simulink model "sim004"  (R2023b)
settings: Solver=FixedStepAuto  StartTime=0.0  StopTime=5  FixedStep=0.001  RelTol=1e-3  EnableMultiTasking=on
values from neighbouring files (symbols this model uses):
  a1 = 40    [FK.m]    (also in IK_Analytical.m = 0.04; IK_MDH.m = 0.04; IK_Position.m = 0.04; IK_Solver.m = 0.04)
  a2 = 275    [FK.m]    (also in IK_Analytical.m = 0.275; IK_MDH.m = 0.275; IK_Position.m = 0.275; IK_Solver.m = 0.275)
  a3 = 25    [FK.m]    (also in IK_Analytical.m = 0.025; IK_MDH.m = 0.025; IK_Position.m = 0.025; IK_Solver.m = 0.025)
  d1 = 342    [FK.m]    (also in IK_Analytical.m = 0.342; IK_MDH.m = 0.342; IK_Position.m = 0.342; IK_Solver.m = 0.342)
  d4 = 280    [FK.m]    (also in IK_Analytical.m = 0.28; IK_MDH.m = 0.28; IK_Position.m = 0.28; IK_Solver.m = 0.28)
  fc1 = 0    [set_mode_parameter.m]
  fc2 = 0    [set_mode_parameter.m]
  fc3 = 0    [set_mode_parameter.m]
  fc4 = 0    [set_mode_parameter.m]
  fc5 = 0    [set_mode_parameter.m]
  fc6 = 0    [set_mode_parameter.m]
  fv1 = 0    [set_mode_parameter.m]
  fv2 = 0    [set_mode_parameter.m]
  fv3 = 0    [set_mode_parameter.m]
  fv4 = 0    [set_mode_parameter.m]
  fv5 = 0    [set_mode_parameter.m]
  fv6 = 0    [set_mode_parameter.m]
  Ia1 = 0    [set_mode_parameter.m]
  Ia2 = 0    [set_mode_parameter.m]
  Ia3 = 0    [set_mode_parameter.m]
  Ia4 = 0    [set_mode_parameter.m]
  Ia5 = 0    [set_mode_parameter.m]
  Ia6 = 0    [set_mode_parameter.m]
  Ic111 = 0    [set_mode_parameter.m]
  Ic112 = 0    [set_mode_parameter.m]
  Ic113 = 0    [set_mode_parameter.m]
  Ic122 = 0    [set_mode_parameter.m]
  Ic123 = 0    [set_mode_parameter.m]
  Ic133 = 1.3676    [set_mode_parameter.m]
  Ic211 = 8.8194    [set_mode_parameter.m]
  Ic212 = 0    [set_mode_parameter.m]
  Ic213 = 0    [set_mode_parameter.m]
  Ic222 = 6.0549    [set_mode_parameter.m]
  Ic223 = 0    [set_mode_parameter.m]
  Ic233 = 0.9569    [set_mode_parameter.m]
  Ic311 = 0.0332    [set_mode_parameter.m]
  Ic312 = 0    [set_mode_parameter.m]
  Ic313 = 0    [set_mode_parameter.m]
  Ic322 = 1.8442    [set_mode_parameter.m]
  Ic323 = 0    [set_mode_parameter.m]
  Ic333 = 1.0560    (= 1.056)    [set_mode_parameter.m]
  Ic411 = 0.1448    [set_mode_parameter.m]
  Ic412 = 0    [set_mode_parameter.m]
  Ic413 = 0    [set_mode_parameter.m]
  Ic422 = 0.0015    [set_mode_parameter.m]
  Ic423 = 0    [set_mode_parameter.m]
  Ic433 = 0.0822    [set_mode_parameter.m]
  Ic511 = 0    [set_mode_parameter.m]
  Ic512 = 0    [set_mode_parameter.m]
  Ic513 = 0    [set_mode_parameter.m]
  Ic522 = 0.0121    [set_mode_parameter.m]
  Ic523 = 0    [set_mode_parameter.m]
  Ic533 = 0.0299    [set_mode_parameter.m]
  Ic611 = 0.0134    [set_mode_parameter.m]
  Ic612 = 0    [set_mode_parameter.m]
  Ic613 = 0    [set_mode_parameter.m]
  Ic622 = 0    [set_mode_parameter.m]
  Ic623 = 0    [set_mode_parameter.m]
  Ic633 = 0.0051    [set_mode_parameter.m]
  m = (c1*px + s1*py) - dt*(c1*ax + s1*ay) - a1    [IK_6DOF_Robot.m]    (also in IK_MDH.m = pwx_1 - a1; IK_MDH_Robot.m = rho - a1)
  m1 = 0.167    [set_mode_parameter.m]
  m2 = 1    [set_mode_parameter.m]
  m3 = 0.5    [set_mode_parameter.m]
  m4 = 0.333    [set_mode_parameter.m]
  m5 = 0.25    [set_mode_parameter.m]
  m6 = 0.2    [set_mode_parameter.m]
  mc11 = 0    [set_mode_parameter.m]
  mc12 = 0    [set_mode_parameter.m]
  mc13 = 0.2    [set_mode_parameter.m]
  mc21 = 0.1291    [set_mode_parameter.m]
  mc22 = 0    [set_mode_parameter.m]
  mc23 = 3.3117    [set_mode_parameter.m]
  mc31 = 1.6484    [set_mode_parameter.m]
  mc32 = 0    [set_mode_parameter.m]
  mc33 = 0.8748    [set_mode_parameter.m]
  mc41 = 0.3200    (= 0.32)    [set_mode_parameter.m]
  mc42 = 0.2324    [set_mode_parameter.m]
  mc43 = 0.7083    [set_mode_parameter.m]
  mc51 = 0.4574    [set_mode_parameter.m]
  mc52 = 0    [set_mode_parameter.m]
  mc53 = 0.6427    [set_mode_parameter.m]
  mc61 = 0.3200    (= 0.32)    [set_mode_parameter.m]
  mc62 = -0.0513    [set_mode_parameter.m]
  mc63 = 0.6417    [set_mode_parameter.m]
  N = size(waypoints, 2)    [run_trajectory.m]
  s = zc - d(1)    [inverse_kinematics_6dof.m]
  XB4 = SerialLink([L1 L2 L3 L4 L5 L6], 'name', 'XB4')    [Toolbox_Motheds_1.m]
undefined symbols (not defined in the file or in its folder): X, Y, Z
libraries: sm_lib x56, nesl_utility x31, simulink x2, simulink_extras x1
(part 1 of 2)
settings Model: Creator=Administrator  LastModifiedBy=jiehuang
settings SolverCC: AlgebraicLoopSolver=TrustRegion
settings DataIOCC: ReturnWorkspaceOutputs=off
settings OptimizationCC: LifeSpan=inf
settings DebuggingCC: UnconnectedInputMsg=warning  UnconnectedOutputMsg=warning  UnconnectedLineMsg=warning  SFUnexpectedBacktrackingDiag=warning  SFNoUnconditionalDefaultTransitionDiag=warning  ArithmeticOperatorsInVariantConditions=warning
settings ModelReferenceCC: EnableRefExpFcnMdlSchedulingChecks=on
settings SFSimCC: SimUseLocalCustomCode=off  CustomCodeUndefinedFunction=UseInterfaceOnly
settings RTWCC: RTWUseLocalCustomCode=off
settings CodeAppCC: StateflowObjectComments=on
settings GRTTargetCC: TargetLangStandard=C89/C90 (ANSI)
settings ConfigComp: CovMetricSettings=dw  CovSaveCumulativeToWorkspaceVar=on  CovSaveSingleToWorkspaceVar=on  CovExternalEMLEnable=off
settings SimscapeCC: SimscapeNormalizeSystem=off

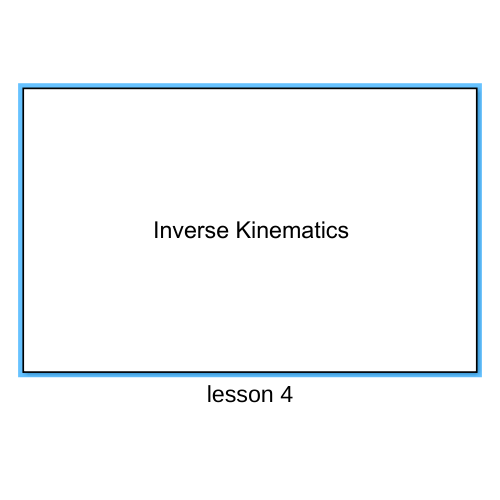
[thumbnail: Simulink's stored preview of the top-level diagram]
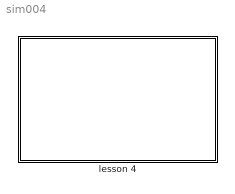
== system sim004 ==
  lesson 4 : Subsystem
      mask Display: disp('Inverse Kinematics')

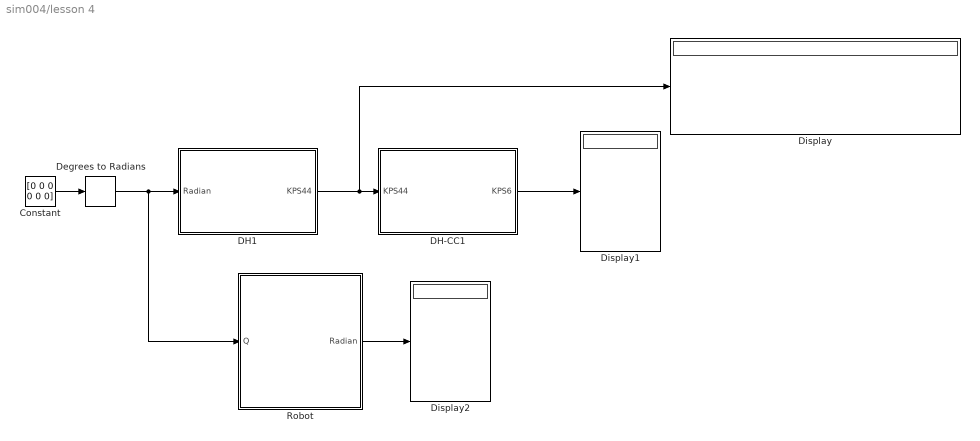
== system sim004/lesson 4 ==
  Constant : Constant  Value=[0 0 0 0 0 0]  VectorParams1D=off
  DH-CC1 : MATLAB Function  TreatAsAtomicUnit=on
  DH1 : MATLAB Function  TreatAsAtomicUnit=on
  Degrees to Radians : simulink_extras/Transformations/Degrees to Radians
  Display : Display
      settings: Decimation=16
  Display1 : Display
      settings: Decimation=6
  Display2 : Display
      settings: Decimation=6
  Robot : Subsystem
  wires:
  DH1/1(KPS44) -> Display/1, DH-CC1/1(KPS44)
  DH-CC1/1(KPS6) -> Display1/1
  Robot/1(Radian) -> Display2/1
  Constant/1 -> Degrees to Radians/1
  Degrees to Radians/1 -> Robot/1(Q), DH1/1(Radian)

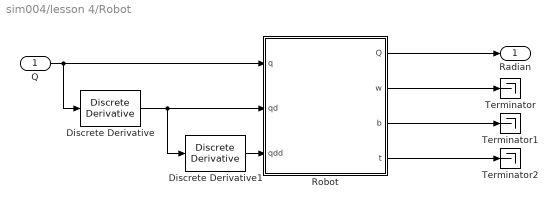
== system sim004/lesson 4/Robot ==
  Q : Inport
  Discrete Derivative : simulink/Discrete/Discrete Derivative  gainval=1.0  ICPrevScaledInput=0.0  OutMin=[]  OutMax=[]  OutDataType=fixdt(1, 16)  OutScaling=2^-10  DoSatur=off
  Discrete Derivative1 : simulink/Discrete/Discrete Derivative  gainval=1.0  ICPrevScaledInput=0.0  OutMin=[]  OutMax=[]  OutDataType=fixdt(1, 16)  OutScaling=2^-10  DoSatur=off
  Robot : Subsystem
  Terminator : Terminator
  Terminator1 : Terminator
  Terminator2 : Terminator
  Radian : Outport
  wires:
  Robot/1(Q) -> Radian/1
  Robot/2(w) -> Terminator/1
  Robot/3(b) -> Terminator1/1
  Robot/4(t) -> Terminator2/1
  Q/1 -> Discrete Derivative/1, Robot/1(q)
  Discrete Derivative/1 -> Discrete Derivative1/1, Robot/2(qd)
  Discrete Derivative1/1 -> Robot/3(qdd)

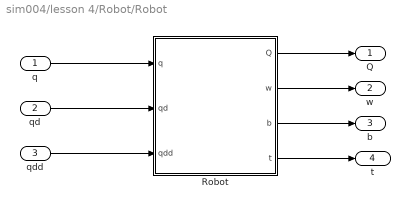
== system sim004/lesson 4/Robot/Robot ==
  q : Inport
  qd : Inport  Port=2
  qdd : Inport  Port=3
  Robot : Subsystem
  Q : Outport
  w : Outport  Port=2
  b : Outport  Port=3
  t : Outport  Port=4
  wires:
  Robot/1(Q) -> Q/1
  Robot/2(w) -> w/1
  Robot/3(b) -> b/1
  Robot/4(t) -> t/1
  q/1 -> Robot/1(q)
  qd/1 -> Robot/2(qd)
  qdd/1 -> Robot/3(qdd)

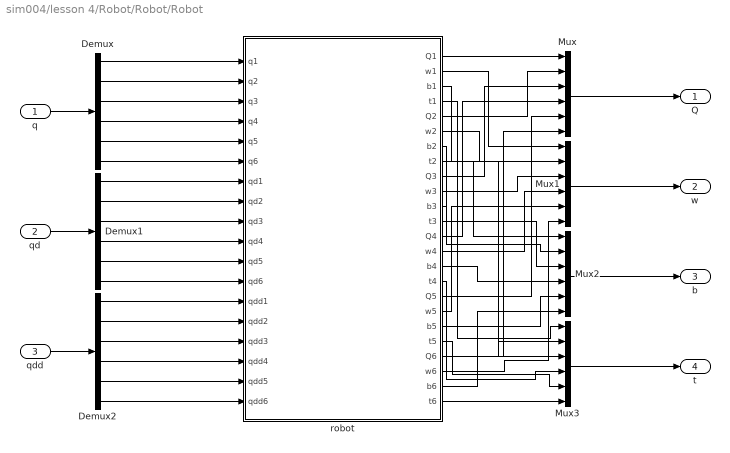
== system sim004/lesson 4/Robot/Robot/Robot ==
  q : Inport
  qd : Inport  Port=2
  qdd : Inport  Port=3
  Demux : Demux  Outputs=6
  Demux1 : Demux  Outputs=6
  Demux2 : Demux  Outputs=6
  Mux{,1..3} (4 alike) : Mux  Inputs=6
  robot : Subsystem
  Q : Outport
  w : Outport  Port=2
  b : Outport  Port=3
  t : Outport  Port=4
  wires:
  q/1 -> Demux/1
  robot/1(Q1) -> Mux/1
  robot/5(Q2) -> Mux/2
  robot/9(Q3) -> Mux/3
  robot/13(Q4) -> Mux/4
  robot/17(Q5) -> Mux/5
  robot/21(Q6) -> Mux/6
  robot/2(w1) -> Mux1/1
  robot/3(b1) -> Mux2/1
  robot/6(w2) -> Mux1/2
  robot/10(w3) -> Mux1/3
  robot/14(w4) -> Mux1/4
  robot/18(w5) -> Mux1/5
  robot/22(w6) -> Mux1/6
  robot/7(b2) -> Mux2/2
  robot/11(b3) -> Mux2/3
  robot/15(b4) -> Mux2/4
  robot/19(b5) -> Mux2/5
  robot/23(b6) -> Mux2/6
  robot/4(t1) -> Mux3/1
  robot/8(t2) -> Mux3/2
  robot/12(t3) -> Mux3/3
  robot/16(t4) -> Mux3/4
  robot/20(t5) -> Mux3/5
  robot/24(t6) -> Mux3/6
  Mux/1 -> Q/1
  Mux1/1 -> w/1
  Mux2/1 -> b/1
  Mux3/1 -> t/1
  Demux/1 -> robot/1(q1)
  Demux/2 -> robot/2(q2)
  Demux/3 -> robot/3(q3)
  Demux/4 -> robot/4(q4)
  Demux/5 -> robot/5(q5)
  Demux/6 -> robot/6(q6)
  Demux1/2 -> robot/8(qd2)
  Demux1/3 -> robot/9(qd3)
  Demux1/4 -> robot/10(qd4)
  Demux1/5 -> robot/11(qd5)
  Demux1/6 -> robot/12(qd6)
  Demux1/1 -> robot/7(qd1)
  qd/1 -> Demux1/1
  Demux2/2 -> robot/14(qdd2)
  Demux2/3 -> robot/15(qdd3)
  Demux2/4 -> robot/16(qdd4)
  Demux2/5 -> robot/17(qdd5)
  Demux2/6 -> robot/18(qdd6)
  Demux2/1 -> robot/13(qdd1)
  qdd/1 -> Demux2/1

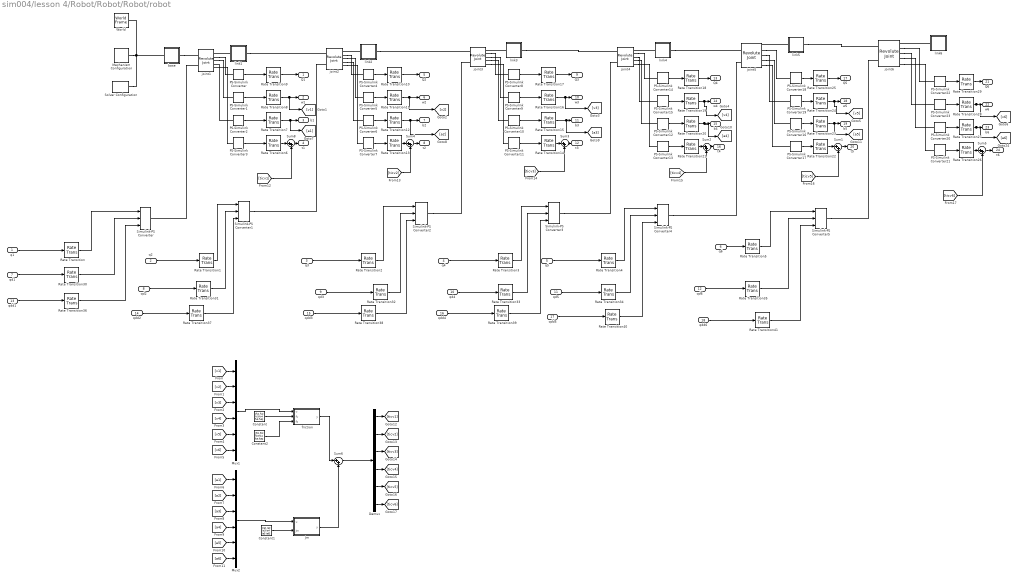
== system sim004/lesson 4/Robot/Robot/Robot/robot ==
  q1 : Inport
  q2 : Inport  Port=2
  q3 : Inport  Port=3
  q4 : Inport  Port=4
  q5 : Inport  Port=5
  q6 : Inport  Port=6
  qd1 : Inport  Port=7
  qd2 : Inport  Port=8
  qd3 : Inport  Port=9
  qd4 : Inport  Port=10
  qd5 : Inport  Port=11
  qd6 : Inport  Port=12
  qdd1 : Inport  Port=13
  qdd2 : Inport  Port=14
  qdd3 : Inport  Port=15
  qdd4 : Inport  Port=16
  qdd5 : Inport  Port=17
  qdd6 : Inport  Port=18
  Constant : Constant  Value=[fv1 fv2 fv3 fv4 fv5 fv6]
  Constant1 : Constant  Value=[Ia1 Ia2 Ia3 Ia4 Ia5 Ia6]
  Constant2 : Constant  Value=[fc1 fc2 fc3 fc4 fc5 fc6]
  Demux : Demux  Outputs=6
  Jm : MATLAB Function  TreatAsAtomicUnit=on
  Mechanism Configuration : sm_lib/Utilities/Mechanism Configuration  UniformGravity=Constant  GravityVector=[0 0 -9.802]  GravityVectorUnits=m/s^2  LinearizationDelta=0.001  JointModeTransitionNonlinearIterations=2
  Mux1 : Mux  Inputs=6
  Mux2 : Mux  Inputs=6
  PS-Simulink Converter{,4,8,14,18,22} (6 alike) : nesl_utility/PS-Simulink Converter  PhysicalDomain=network_engine_domain  SubClassName=ps_output  LeftPortType=input  RightPortType=output  PseudoPeriodic=off  Frequencies=[]  VectorFormat=1-D array  Unit=rad  AffineConversion=off
  PS-Simulink Converter{1,5,9,15,19,23} (6 alike) : nesl_utility/PS-Simulink Converter  PhysicalDomain=network_engine_domain  SubClassName=ps_output  LeftPortType=input  RightPortType=output  PseudoPeriodic=off  Frequencies=[]  VectorFormat=1-D array  Unit=rad/s  AffineConversion=off
  PS-Simulink Converter{2,6,10,12,16,20} (6 alike) : nesl_utility/PS-Simulink Converter  PhysicalDomain=network_engine_domain  SubClassName=ps_output  LeftPortType=input  RightPortType=output  PseudoPeriodic=off  Frequencies=[]  VectorFormat=1-D array  Unit=1  AffineConversion=off
  PS-Simulink Converter{3,7,11,13,17,21} (6 alike) : nesl_utility/PS-Simulink Converter  PhysicalDomain=network_engine_domain  SubClassName=ps_output  LeftPortType=input  RightPortType=output  PseudoPeriodic=off  Frequencies=[]  VectorFormat=1-D array  Unit=N*m  AffineConversion=off
  Rate Transition{,1..41} (42 alike) : RateTransition
  Simulink-PS Converter{,1..5} (6 alike) : nesl_utility/Simulink-PS Converter  PhysicalDomain=network_engine_domain  SubClassName=ps_input  LeftPortType=input  RightPortType=output  PseudoPeriodic=off  Frequencies=[]  NoiseDistribution=none  NoiseParameters=[]  Unit=rad  AffineConversion=off  FilteringAndDerivatives=provide  SimscapeFilterOrder=1  InputFilterTimeConstant=0.001  UdotUserProvided=2
  Solver Configuration : nesl_utility/Solver Configuration  PhysicalDomain=network_engine_domain  SubClassName=solver  LeftPortType=input  RightPortType=generic  Tones=[]  Harmonics=[]  SimulateNoise=off  Profile=off  UseLocalSampling=off  EnableSwitchedLinearOptims=on  FrequencyDomain=off  UseCCode=off  RelTol=0.001  AbsTol=1e-06  MinStep=1e-09  ToWorkspace=off  RevertToSquareIcSolve=off  NumHomotopyIterations=100  PhasorMode=off  PhasorModeNumHarmonics=1  ConsistencySolver=NEWTON_FTOL  IndexReductionMethod=DerivativeReplacement  DoDC=off  ResidualTolerance=1e-09  ConsistencyTolSource=GLOBAL  ConsistencyAbsTol=0.001  ConsistencyRelTol=0.001  ConsistencyTolFactor=0.001  UseLocalSolver=off  LocalSolverChoice=NE_BACKWARD_EULER_ADVANCER  ResolveIndetEquations=on  FunctionEvalNumThread=1  LocalSolverSampleTime=0.001  DoFixedCost=off  MaxNonlinIter=3  MaxModeIter=2  ComputeImpulses=off  ImpulseIterations=2  LinearAlgebra=Sparse  LinearAlgebraNumThread=0  EquationFormulation=NE_TIME_EF  DelaysMemoryBudget=1024  AutomaticFiltering=on  FilteringTimeConstant=0.001  PartitionStorageMethod=AS_NEEDED  PartitionMemoryBudget=1024  PartitionMethod=FAST  MultibodyUseLocalSolver=off  MultibodyLocalSolverChoice=ODE1  MultibodyLocalSolverSampleTime=0.001
  Sum{1..6,8} (7 alike) : Sum  Inputs=|++
  World : sm_lib/Frames and Transforms/World Frame
  base : Subsystem
  friction : MATLAB Function  TreatAsAtomicUnit=on
  joint1 : sm_lib/Joints/Revolute Joint  JointMode=Normal  SenseConstraintForce=off  SenseConstraintForceX=off  SenseConstraintForceY=off  SenseConstraintForceZ=off  SenseConstraintTorque=off  SenseConstraintTorqueX=off  SenseConstraintTorqueY=off  SenseConstraintTorqueZ=off  SenseTotalForce=off  SenseTotalForceX=off  SenseTotalForceY=off  SenseTotalForceZ=off  SenseTotalTorque=off  SenseTotalTorqueX=off  SenseTotalTorqueY=off  SenseTotalTorqueZ=off  CompositeWrenchDir=FollowerOnBase  CompositeWrenchFrame=FollowerFrame  EquilibriumPosition=0  EquilibriumPositionUnits=deg  SpringStiffness=0  SpringStiffnessUnits=N*m/deg  DampingCoefficient=0  DampingCoefficientUnits=N*m/(deg/s)  TorqueActuationMode=ComputedTorque  MotionActuationMode=InputMotion  SensePosition=on  SenseVelocity=on  SenseAcceleration=on  SenseTorqueForce=on  SenseLowerLimitTorqueForce=off  SenseUpperLimitTorqueForce=off  LowerLimitSpecify=off  LowerLimitBound=-90  LowerLimitBoundUnits=deg  LowerLimitStiffness=1e4  LowerLimitStiffnessUnits=N*m/deg  LowerLimitDamping=10  LowerLimitDampingUnits=N*m/(deg/s)  LowerLimitTransitionRegionWidth=0.1  LowerLimitTransitionRegionWidthUnits=deg  UpperLimitSpecify=off  UpperLimitBound=90  UpperLimitBoundUnits=deg  UpperLimitStiffness=1e4  UpperLimitStiffnessUnits=N*m/deg  UpperLimitDamping=10  UpperLimitDampingUnits=N*m/(deg/s)  UpperLimitTransitionRegionWidth=0.1  UpperLimitTransitionRegionWidthUnits=deg  PositionTargetSpecify=off  PositionTargetPriority=High  PositionTargetValue=0  PositionTargetValueUnits=deg  VelocityTargetSpecify=off  VelocityTargetPriority=High  VelocityTargetValue=0  VelocityTargetValueUnits=deg/s
  joint{2..6} (5 alike) : sm_lib/Joints/Revolute Joint  JointMode=Normal  SenseConstraintForce=off  SenseConstraintForceX=off  SenseConstraintForceY=off  SenseConstraintForceZ=off  SenseConstraintTorque=off  SenseConstraintTorqueX=off  SenseConstraintTorqueY=off  SenseConstraintTorqueZ=off  SenseTotalForce=off  SenseTotalForceX=off  SenseTotalForceY=off  SenseTotalForceZ=off  SenseTotalTorque=off  SenseTotalTorqueX=off  SenseTotalTorqueY=off  SenseTotalTorqueZ=off  CompositeWrenchDir=FollowerOnBase  CompositeWrenchFrame=BaseFrame  EquilibriumPosition=0  EquilibriumPositionUnits=deg  SpringStiffness=0  SpringStiffnessUnits=N*m/deg  DampingCoefficient=0  DampingCoefficientUnits=N*m/(deg/s)  TorqueActuationMode=ComputedTorque  MotionActuationMode=InputMotion  SensePosition=on  SenseVelocity=on  SenseAcceleration=on  SenseTorqueForce=on  SenseLowerLimitTorqueForce=off  SenseUpperLimitTorqueForce=off  LowerLimitSpecify=off  LowerLimitBound=-90  LowerLimitBoundUnits=deg  LowerLimitStiffness=1e4  LowerLimitStiffnessUnits=N*m/deg  LowerLimitDamping=10  LowerLimitDampingUnits=N*m/(deg/s)  LowerLimitTransitionRegionWidth=0.1  LowerLimitTransitionRegionWidthUnits=deg  UpperLimitSpecify=off  UpperLimitBound=90  UpperLimitBoundUnits=deg  UpperLimitStiffness=1e4  UpperLimitStiffnessUnits=N*m/deg  UpperLimitDamping=10  UpperLimitDampingUnits=N*m/(deg/s)  UpperLimitTransitionRegionWidth=0.1  UpperLimitTransitionRegionWidthUnits=deg  PositionTargetSpecify=off  PositionTargetPriority=High  PositionTargetValue=0  PositionTargetValueUnits=deg  VelocityTargetSpecify=off  VelocityTargetPriority=High  VelocityTargetValue=0  VelocityTargetValueUnits=deg/s
  link1 : Subsystem
  link2 : Subsystem
  link3 : Subsystem
  link4 : Subsystem
  link5 : Subsystem
  link6 : Subsystem
  Q1 : Outport
  w1 : Outport  Port=2
  b1 : Outport  Port=3
  t1 : Outport  Port=4
  Q2 : Outport  Port=5
  w2 : Outport  Port=6
  b2 : Outport  Port=7
  t2 : Outport  Port=8
  Q3 : Outport  Port=9
  w3 : Outport  Port=10
  b3 : Outport  Port=11
  t3 : Outport  Port=12
  Q4 : Outport  Port=13
  w4 : Outport  Port=14
  b4 : Outport  Port=15
  t4 : Outport  Port=16
  Q5 : Outport  Port=17
  w5 : Outport  Port=18
  b5 : Outport  Port=19
  t5 : Outport  Port=20
  Q6 : Outport  Port=21
  w6 : Outport  Port=22
  b6 : Outport  Port=23
  t6 : Outport  Port=24
  wires:
  PS-Simulink Converter/1 -> Rate Transition9/1
  PS-Simulink Converter1/1 -> Rate Transition8/1
  PS-Simulink Converter2/1 -> Rate Transition7/1
  PS-Simulink Converter3/1 -> Rate Transition6/1
  PS-Simulink Converter7/1 -> Rate Transition13/1
  PS-Simulink Converter18/1 -> Rate Transition25/1
  PS-Simulink Converter5/1 -> Rate Transition11/1
  PS-Simulink Converter6/1 -> Rate Transition12/1
  PS-Simulink Converter4/1 -> Rate Transition10/1
  PS-Simulink Converter8/1 -> Rate Transition17/1
  PS-Simulink Converter9/1 -> Rate Transition16/1
  PS-Simulink Converter10/1 -> Rate Transition15/1
  PS-Simulink Converter11/1 -> Rate Transition14/1
  PS-Simulink Converter14/1 -> Rate Transition18/1
  PS-Simulink Converter15/1 -> Rate Transition19/1
  PS-Simulink Converter12/1 -> Rate Transition20/1
  PS-Simulink Converter13/1 -> Rate Transition21/1
  PS-Simulink Converter19/1 -> Rate Transition24/1
  PS-Simulink Converter16/1 -> Rate Transition23/1
  PS-Simulink Converter17/1 -> Rate Transition22/1
  PS-Simulink Converter22/1 -> Rate Transition29/1
  PS-Simulink Converter23/1 -> Rate Transition28/1
  PS-Simulink Converter20/1 -> Rate Transition27/1
  PS-Simulink Converter21/1 -> Rate Transition26/1
  Rate Transition1/1 -> Simulink-PS Converter1/1
  Rate Transition2/1 -> Simulink-PS Converter2/1
  Rate Transition3/1 -> Simulink-PS Converter3/1
  Rate Transition4/1 -> Simulink-PS Converter4/1
  Rate Transition5/1 -> Simulink-PS Converter5/1
  Rate Transition/1 -> Simulink-PS Converter/1
  Rate Transition7/1 -> [a1], b1/1
  Rate Transition8/1 -> [v1], w1/1
  Rate Transition9/1 -> Q1/1
  Rate Transition10/1 -> Q2/1
  Rate Transition11/1 -> [v2], w2/1
  Rate Transition12/1 -> [a2], b2/1
  Rate Transition15/1 -> [a3], b3/1
  Rate Transition16/1 -> [v3], w3/1
  Rate Transition17/1 -> Q3/1
  Rate Transition18/1 -> Q4/1
  Rate Transition19/1 -> [v4], w4/1
  Rate Transition20/1 -> [a4], b4/1
  Rate Transition23/1 -> [a5], b5/1
  Rate Transition24/1 -> [v5], w5/1
  Rate Transition25/1 -> Q5/1
  Rate Transition27/1 -> [a6], b6/1
  Rate Transition28/1 -> [v6], w6/1
  Rate Transition29/1 -> Q6/1
  [v1] -> Mux1/1
  [v2] -> Mux1/2
  [v3] -> Mux1/3
  [v4] -> Mux1/4
  [v5] -> Mux1/5
  [v6] -> Mux1/6
  [a1] -> Mux2/1
  [a2] -> Mux2/2
  [a3] -> Mux2/3
  [a5] -> Mux2/5
  [a4] -> Mux2/4
  [a6] -> Mux2/6
  Demux/1 -> [ticv1]
  Demux/2 -> [ticv2]
  Demux/3 -> [ticv3]
  Demux/4 -> [ticv4]
  Demux/5 -> [ticv5]
  Demux/6 -> [ticv6]
  [ticv1] -> Sum8/2
  [ticv3] -> Sum3/2
  [ticv4] -> Sum2/2
  [ticv5] -> Sum1/2
  [ticv6] -> Sum5/2
  Mux1/1 -> friction/1(u)
  Mux2/1 -> Jm/1(u)
  friction/1(y) -> Sum6/1
  Jm/1(y) -> Sum6/2
  Constant/1 -> friction/2(fv)
  Constant1/1 -> Jm/2(Jm)
  Constant2/1 -> friction/3(fc)
  Sum6/1 -> Demux/1
  q1/1 -> Rate Transition/1
  q2/1 -> Rate Transition1/1
  q3/1 -> Rate Transition2/1
  q4/1 -> Rate Transition3/1
  q5/1 -> Rate Transition4/1
  q6/1 -> Rate Transition5/1
  Rate Transition26/1 -> Sum5/1
  Sum5/1 -> t6/1
  Rate Transition22/1 -> Sum1/1
  Sum1/1 -> t5/1
  Rate Transition21/1 -> Sum2/1
  Sum2/1 -> t4/1
  Rate Transition14/1 -> Sum3/1
  Sum3/1 -> t3/1
  Rate Transition13/1 -> Sum4/1
  Sum4/1 -> t2/1
  [ticv2] -> Sum4/2
  Sum8/1 -> t1/1
  Rate Transition6/1 -> Sum8/1
  qd1/1 -> Rate Transition30/1
  Rate Transition30/1 -> Simulink-PS Converter/2
  qd2/1 -> Rate Transition31/1
  Rate Transition31/1 -> Simulink-PS Converter1/2
  qd3/1 -> Rate Transition32/1
  Rate Transition32/1 -> Simulink-PS Converter2/2
  qd4/1 -> Rate Transition33/1
  Rate Transition33/1 -> Simulink-PS Converter3/2
  qd5/1 -> Rate Transition34/1
  Rate Transition34/1 -> Simulink-PS Converter4/2
  qd6/1 -> Rate Transition35/1
  Rate Transition35/1 -> Simulink-PS Converter5/2
  qdd1/1 -> Rate Transition36/1
  Rate Transition36/1 -> Simulink-PS Converter/3
  qdd2/1 -> Rate Transition37/1
  Rate Transition37/1 -> Simulink-PS Converter1/3
  qdd3/1 -> Rate Transition38/1
  Rate Transition38/1 -> Simulink-PS Converter2/3
  qdd4/1 -> Rate Transition39/1
  Rate Transition39/1 -> Simulink-PS Converter3/3
  qdd5/1 -> Rate Transition40/1
  Rate Transition40/1 -> Simulink-PS Converter4/3
  qdd6/1 -> Rate Transition41/1
  Rate Transition41/1 -> Simulink-PS Converter5/3
  connections:
  link6/LConn1 -- joint6/RConn1
  link5/RConn1 -- joint6/LConn1
  link2/LConn1 -- joint2/RConn1
  link1/RConn1 -- joint2/LConn1
  base/RConn1 -- joint1/LConn1
  link1/LConn1 -- joint1/RConn1
  link2/RConn1 -- joint3/LConn1
  link3/LConn1 -- joint3/RConn1
  link4/LConn1 -- joint4/RConn1
  link4/RConn1 -- joint5/LConn1
  link5/LConn1 -- joint5/RConn1
  link3/RConn1 -- joint4/LConn1
  base/LConn1 -- Mechanism Configuration/RConn1 -- Solver Configuration/RConn1 -- World/RConn1
  Simulink-PS Converter1/RConn1 -- joint2/LConn2
  Simulink-PS Converter2/RConn1 -- joint3/LConn2
  Simulink-PS Converter3/RConn1 -- joint4/LConn2
  Simulink-PS Converter4/RConn1 -- joint5/LConn2
  Simulink-PS Converter5/RConn1 -- joint6/LConn2
  joint1/RConn2 -- PS-Simulink Converter/LConn1
  joint1/RConn3 -- PS-Simulink Converter1/LConn1
  PS-Simulink Converter2/LConn1 -- joint1/RConn4
  joint1/RConn5 -- PS-Simulink Converter3/LConn1
  joint2/RConn2 -- PS-Simulink Converter4/LConn1
  joint2/RConn3 -- PS-Simulink Converter5/LConn1
  joint2/RConn4 -- PS-Simulink Converter6/LConn1
  joint2/RConn5 -- PS-Simulink Converter7/LConn1
  joint3/RConn2 -- PS-Simulink Converter8/LConn1
  joint3/RConn3 -- PS-Simulink Converter9/LConn1
  joint3/RConn4 -- PS-Simulink Converter10/LConn1
  joint3/RConn5 -- PS-Simulink Converter11/LConn1
  joint4/RConn2 -- PS-Simulink Converter14/LConn1
  joint4/RConn3 -- PS-Simulink Converter15/LConn1
  joint4/RConn4 -- PS-Simulink Converter12/LConn1
  joint4/RConn5 -- PS-Simulink Converter13/LConn1
  joint5/RConn2 -- PS-Simulink Converter18/LConn1
  joint5/RConn3 -- PS-Simulink Converter19/LConn1
  joint5/RConn4 -- PS-Simulink Converter16/LConn1
  joint5/RConn5 -- PS-Simulink Converter17/LConn1
  joint6/RConn2 -- PS-Simulink Converter22/LConn1
  joint6/RConn3 -- PS-Simulink Converter23/LConn1
  joint6/RConn4 -- PS-Simulink Converter20/LConn1
  joint6/RConn5 -- PS-Simulink Converter21/LConn1
  joint1/LConn2 -- Simulink-PS Converter/RConn1

== system sim004/lesson 4/Robot/Robot/Robot/robot/base ==
  Inertia : sm_lib/Body Elements/Inertia  InertiaType=Custom  Mass=1  MassUnits=kg  CenterOfMass=[0 0 0]  CenterOfMassUnits=m  MomentsOfInertia=[1 1 1]  MomentsOfInertiaUnits=kg*m^2  ProductsOfInertia=[0 0 0]  ProductsOfInertiaUnits=kg*m^2  GraphicType=Marker  MarkerShape=Inertia  MarkerSize=20  GraphicVisPropType=SimpleVisualProperties  GraphicDiffuseColor=[0.5 0.5 0.5]  GraphicSpecularColor=[0.5 0.5 0.5 1.0]  GraphicAmbientColor=[0.15 0.15 0.15 1.0]  GraphicEmissiveColor=[0.0 0.0 0.0 1.0]  GraphicShininess=75  GraphicOpacity=1.0
  Reference Frame : sm_lib/Frames and Transforms/Reference Frame
  base : sm_lib/Body Elements/File Solid  ExtGeomFileName=/home/jiehuang/Documents/Custom-Robot/Matlab_Study/Matlab2023Project/IntroductionBook/程序/XB4模型/XB4-base.STL  UnitType=Custom  ExtGeomFileUnits=mm  StepReaderType=HEX  ExportConvexHullGeometry=off  InertiaType=Custom  Mass=0  MassUnits=kg  CenterOfMass=[0 0 0]  CenterOfMassUnits=m  MomentsOfInertia=[0 0 0 ]  MomentsOfInertiaUnits=kg*m^2  ProductsOfInertia=[0 0 0]  ProductsOfInertiaUnits=kg*m^2  BasedOnType=Density  Density=1000  DensityUnits=kg/(m^3)  DoExposeReferenceFrame=on  SerializedFrames=<Frames/>  GraphicType=FromGeometry  MarkerShape=Sphere  MarkerSize=10  GraphicVisPropType=SimpleVisualProperties  GraphicDiffuseColor=[0.5 0.5 0.5]  GraphicSpecularColor=[0.5 0.5 0.5 1.0]  GraphicAmbientColor=[0.15 0.15 0.15 1.0]  GraphicEmissiveColor=[0.0 0.0 0.0 1.0]  GraphicShininess=75  GraphicOpacity=1.0
  joint1_OriginTransform1 : sm_lib/Frames and Transforms/Rigid Transform  TranslationMethod=Cartesian  TranslationStandardOffset=0  TranslationStandardOffsetUnits=m  TranslationStandardAxis=+Z  TranslationCartesianOffset=[0 0 d1]  TranslationCartesianOffsetUnits=m  TranslationROffset=0  TranslationROffsetUnits=m  TranslationZOffset=0  TranslationZOffsetUnits=m  TranslationThetaOffset=0  TranslationThetaOffsetUnits=deg  RotationMethod=RotationSequence  RotationAngleUnits=deg  RotationStandardAxis=+Z  RotationAngle=0.0  RotationArbitraryAxis=[0 0 1]  FollAlignAxisA=+X  BaseAlignAxisA=+Y  FollAlignAxisB=+Y  BaseAlignAxisB=+Z  RotationSequenceAxes=BaseAxes  RotationSequence=XYZ  RotationSequenceAngles=[0 0 0]  RotationSequenceAnglesUnits=rad  RotationMatrix=[1 0 0; 0 1 0; 0 0 1]  Quaternion=[1 0 0 0]
  F : PMIOPort  Side=Left
  F1 : PMIOPort  Port=2  Side=Right
  connections:
  Reference Frame/RConn1 -- base/RConn1 -- Inertia/RConn1 -- joint1_OriginTransform1/LConn1 -- F/RConn1
  F1/RConn1 -- joint1_OriginTransform1/RConn1

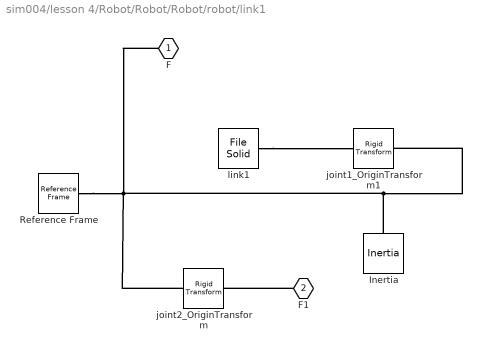
== system sim004/lesson 4/Robot/Robot/Robot/robot/link1 ==
  Inertia : sm_lib/Body Elements/Inertia  InertiaType=Custom  Mass=m1  MassUnits=kg  CenterOfMass=[mc11 mc12 mc13]  CenterOfMassUnits=m  MomentsOfInertia=[Ic111 Ic122 Ic133]  MomentsOfInertiaUnits=kg*m^2  ProductsOfInertia=[Ic123 Ic113 Ic112]  ProductsOfInertiaUnits=kg*m^2  GraphicType=Marker  MarkerShape=Inertia  MarkerSize=20  GraphicVisPropType=SimpleVisualProperties  GraphicDiffuseColor=[0.5 0.5 0.5]  GraphicSpecularColor=[0.5 0.5 0.5 1.0]  GraphicAmbientColor=[0.15 0.15 0.15 1.0]  GraphicEmissiveColor=[0.0 0.0 0.0 1.0]  GraphicShininess=75  GraphicOpacity=1.0
  Reference Frame : sm_lib/Frames and Transforms/Reference Frame
  joint1_OriginTransform1 : sm_lib/Frames and Transforms/Rigid Transform  TranslationMethod=Cartesian  TranslationStandardOffset=0  TranslationStandardOffsetUnits=m  TranslationStandardAxis=+Z  TranslationCartesianOffset=[0 0 d1]  TranslationCartesianOffsetUnits=m  TranslationROffset=0  TranslationROffsetUnits=m  TranslationZOffset=0  TranslationZOffsetUnits=m  TranslationThetaOffset=0  TranslationThetaOffsetUnits=deg  RotationMethod=RotationSequence  RotationAngleUnits=deg  RotationStandardAxis=+Z  RotationAngle=0.0  RotationArbitraryAxis=[0 0 1]  FollAlignAxisA=+X  BaseAlignAxisA=+Y  FollAlignAxisB=+Y  BaseAlignAxisB=+Z  RotationSequenceAxes=BaseAxes  RotationSequence=XYZ  RotationSequenceAngles=[0 0 0]  RotationSequenceAnglesUnits=rad  RotationMatrix=[1 0 0; 0 1 0; 0 0 1]  Quaternion=[1 0 0 0]
  joint2_OriginTransform : sm_lib/Frames and Transforms/Rigid Transform  TranslationMethod=Cartesian  TranslationStandardOffset=0  TranslationStandardOffsetUnits=m  TranslationStandardAxis=+Z  TranslationCartesianOffset=[a1 0 0]  TranslationCartesianOffsetUnits=m  TranslationROffset=0  TranslationROffsetUnits=m  TranslationZOffset=0  TranslationZOffsetUnits=m  TranslationThetaOffset=0  TranslationThetaOffsetUnits=deg  RotationMethod=RotationSequence  RotationAngleUnits=deg  RotationStandardAxis=+Z  RotationAngle=0.0  RotationArbitraryAxis=[0 0 1]  FollAlignAxisA=+X  BaseAlignAxisA=+Y  FollAlignAxisB=+Y  BaseAlignAxisB=+Z  RotationSequenceAxes=FollowerAxes  RotationSequence=XYZ  RotationSequenceAngles=[-pi/2 0 -pi/2]  RotationSequenceAnglesUnits=rad  RotationMatrix=[1 0 0; 0 1 0; 0 0 1]  Quaternion=[1 0 0 0]
  link1 : sm_lib/Body Elements/File Solid  ExtGeomFileName=/home/jiehuang/Documents/Custom-Robot/Matlab_Study/Matlab2023Project/IntroductionBook/程序/XB4模型/XB4-1.STL  UnitType=Custom  ExtGeomFileUnits=mm  StepReaderType=HEX  ExportConvexHullGeometry=off  InertiaType=Custom  Mass=0  MassUnits=kg  CenterOfMass=[0 0 0]  CenterOfMassUnits=m  MomentsOfInertia=[0 0 0 ]  MomentsOfInertiaUnits=kg*m^2  ProductsOfInertia=[0 0 0]  ProductsOfInertiaUnits=kg*m^2  BasedOnType=Density  Density=1000  DensityUnits=kg/(m^3)  DoExposeReferenceFrame=on  SerializedFrames=<Frames/>  GraphicType=FromGeometry  MarkerShape=Sphere  MarkerSize=10  GraphicVisPropType=SimpleVisualProperties  GraphicDiffuseColor=[0.5 0.5 0.5]  GraphicSpecularColor=[0.5 0.5 0.5 1.0]  GraphicAmbientColor=[0.15 0.15 0.15 1.0]  GraphicEmissiveColor=[0.0 0.0 0.0 1.0]  GraphicShininess=75  GraphicOpacity=1.0
  F : PMIOPort  Side=Left
  F1 : PMIOPort  Port=2  Side=Right
  connections:
  Reference Frame/RConn1 -- joint1_OriginTransform1/RConn1 -- Inertia/RConn1 -- F/RConn1 -- joint2_OriginTransform/LConn1
  F1/RConn1 -- joint2_OriginTransform/RConn1
  link1/RConn1 -- joint1_OriginTransform1/LConn1

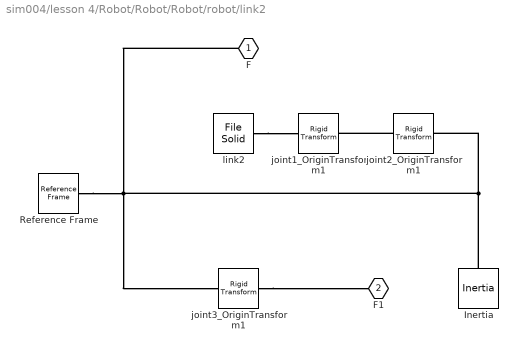
== system sim004/lesson 4/Robot/Robot/Robot/robot/link2 ==
  Inertia : sm_lib/Body Elements/Inertia  InertiaType=Custom  Mass=m2  MassUnits=kg  CenterOfMass=[mc21 mc22 mc23]  CenterOfMassUnits=m  MomentsOfInertia=[Ic211 Ic222 Ic233]  MomentsOfInertiaUnits=kg*m^2  ProductsOfInertia=[Ic223 Ic213 Ic212]  ProductsOfInertiaUnits=kg*m^2  GraphicType=Marker  MarkerShape=Inertia  MarkerSize=20  GraphicVisPropType=SimpleVisualProperties  GraphicDiffuseColor=[0.5 0.5 0.5]  GraphicSpecularColor=[0.5 0.5 0.5 1.0]  GraphicAmbientColor=[0.15 0.15 0.15 1.0]  GraphicEmissiveColor=[0.0 0.0 0.0 1.0]  GraphicShininess=75  GraphicOpacity=1.0
  Reference Frame : sm_lib/Frames and Transforms/Reference Frame
  joint1_OriginTransform1 : sm_lib/Frames and Transforms/Rigid Transform  TranslationMethod=Cartesian  TranslationStandardOffset=0  TranslationStandardOffsetUnits=m  TranslationStandardAxis=+Z  TranslationCartesianOffset=[0 0 d1]  TranslationCartesianOffsetUnits=m  TranslationROffset=0  TranslationROffsetUnits=m  TranslationZOffset=0  TranslationZOffsetUnits=m  TranslationThetaOffset=0  TranslationThetaOffsetUnits=deg  RotationMethod=RotationSequence  RotationAngleUnits=deg  RotationStandardAxis=+Z  RotationAngle=0.0  RotationArbitraryAxis=[0 0 1]  FollAlignAxisA=+X  BaseAlignAxisA=+Y  FollAlignAxisB=+Y  BaseAlignAxisB=+Z  RotationSequenceAxes=BaseAxes  RotationSequence=XYZ  RotationSequenceAngles=[0 0 0]  RotationSequenceAnglesUnits=rad  RotationMatrix=[1 0 0; 0 1 0; 0 0 1]  Quaternion=[1 0 0 0]
  joint2_OriginTransform1 : sm_lib/Frames and Transforms/Rigid Transform  TranslationMethod=Cartesian  TranslationStandardOffset=0  TranslationStandardOffsetUnits=m  TranslationStandardAxis=+Z  TranslationCartesianOffset=[a1 0 0]  TranslationCartesianOffsetUnits=m  TranslationROffset=0  TranslationROffsetUnits=m  TranslationZOffset=0  TranslationZOffsetUnits=m  TranslationThetaOffset=0  TranslationThetaOffsetUnits=deg  RotationMethod=RotationSequence  RotationAngleUnits=deg  RotationStandardAxis=+Z  RotationAngle=0.0  RotationArbitraryAxis=[0 0 1]  FollAlignAxisA=+X  BaseAlignAxisA=+Y  FollAlignAxisB=+Y  BaseAlignAxisB=+Z  RotationSequenceAxes=FollowerAxes  RotationSequence=XYZ  RotationSequenceAngles=[-pi/2 0 -pi/2]  RotationSequenceAnglesUnits=rad  RotationMatrix=[1 0 0; 0 1 0; 0 0 1]  Quaternion=[1 0 0 0]
  joint3_OriginTransform1 : sm_lib/Frames and Transforms/Rigid Transform  TranslationMethod=Cartesian  TranslationStandardOffset=0  TranslationStandardOffsetUnits=m  TranslationStandardAxis=+Z  TranslationCartesianOffset=[a2 0 0]  TranslationCartesianOffsetUnits=m  TranslationROffset=0  TranslationROffsetUnits=m  TranslationZOffset=0  TranslationZOffsetUnits=m  TranslationThetaOffset=0  TranslationThetaOffsetUnits=deg  RotationMethod=RotationSequence  RotationAngleUnits=deg  RotationStandardAxis=+Z  RotationAngle=0.0  RotationArbitraryAxis=[0 0 1]  FollAlignAxisA=+X  BaseAlignAxisA=+Y  FollAlignAxisB=+Y  BaseAlignAxisB=+Z  RotationSequenceAxes=FollowerAxes  RotationSequence=XYZ  RotationSequenceAngles=[0 0 0]  RotationSequenceAnglesUnits=rad  RotationMatrix=[1 0 0; 0 1 0; 0 0 1]  Quaternion=[1 0 0 0]
  link2 : sm_lib/Body Elements/File Solid  ExtGeomFileName=/home/jiehuang/Documents/Custom-Robot/Matlab_Study/Matlab2023Project/IntroductionBook/程序/XB4模型/XB4-2.STL  UnitType=Custom  ExtGeomFileUnits=mm  StepReaderType=HEX  ExportConvexHullGeometry=off  InertiaType=Custom  Mass=0  MassUnits=kg  CenterOfMass=[0 0 0]  CenterOfMassUnits=m  MomentsOfInertia=[0 0 0]  MomentsOfInertiaUnits=kg*m^2  ProductsOfInertia=[0 0 0]  ProductsOfInertiaUnits=kg*m^2  BasedOnType=Density  Density=1000  DensityUnits=kg/(m^3)  DoExposeReferenceFrame=on  SerializedFrames=<Frames/>  GraphicType=FromGeometry  MarkerShape=Sphere  MarkerSize=10  GraphicVisPropType=SimpleVisualProperties  GraphicDiffuseColor=[0.5 0.5 0.5]  GraphicSpecularColor=[0.5 0.5 0.5 1.0]  GraphicAmbientColor=[0.15 0.15 0.15 1.0]  GraphicEmissiveColor=[0.0 0.0 0.0 1.0]  GraphicShininess=75  GraphicOpacity=1.0
  F : PMIOPort  Side=Left
  F1 : PMIOPort  Port=2  Side=Right
  connections:
  Reference Frame/RConn1 -- joint2_OriginTransform1/RConn1 -- Inertia/RConn1 -- F/RConn1 -- joint3_OriginTransform1/LConn1
  joint3_OriginTransform1/RConn1 -- F1/RConn1
  joint2_OriginTransform1/LConn1 -- joint1_OriginTransform1/RConn1
  link2/RConn1 -- joint1_OriginTransform1/LConn1

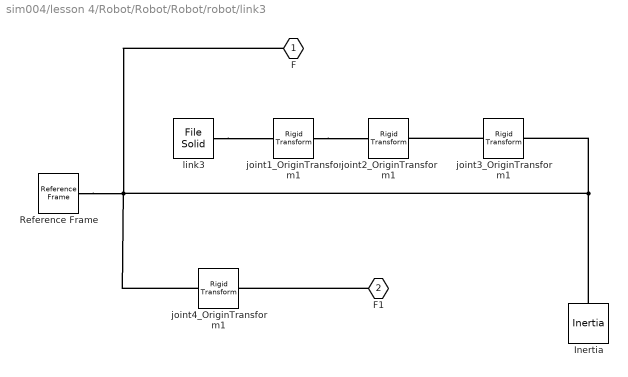
== system sim004/lesson 4/Robot/Robot/Robot/robot/link3 ==
  Inertia : sm_lib/Body Elements/Inertia  InertiaType=Custom  Mass=m3  MassUnits=kg  CenterOfMass=[mc31 mc32 mc33]  CenterOfMassUnits=m  MomentsOfInertia=[Ic311 Ic322 Ic333]  MomentsOfInertiaUnits=kg*m^2  ProductsOfInertia=[Ic323 Ic313 Ic312]  ProductsOfInertiaUnits=kg*m^2  GraphicType=Marker  MarkerShape=Inertia  MarkerSize=20  GraphicVisPropType=SimpleVisualProperties  GraphicDiffuseColor=[0.5 0.5 0.5]  GraphicSpecularColor=[0.5 0.5 0.5 1.0]  GraphicAmbientColor=[0.15 0.15 0.15 1.0]  GraphicEmissiveColor=[0.0 0.0 0.0 1.0]  GraphicShininess=75  GraphicOpacity=1.0
  Reference Frame : sm_lib/Frames and Transforms/Reference Frame
  joint1_OriginTransform1 : sm_lib/Frames and Transforms/Rigid Transform  TranslationMethod=Cartesian  TranslationStandardOffset=0  TranslationStandardOffsetUnits=m  TranslationStandardAxis=+Z  TranslationCartesianOffset=[0 0 d1]  TranslationCartesianOffsetUnits=m  TranslationROffset=0  TranslationROffsetUnits=m  TranslationZOffset=0  TranslationZOffsetUnits=m  TranslationThetaOffset=0  TranslationThetaOffsetUnits=deg  RotationMethod=RotationSequence  RotationAngleUnits=deg  RotationStandardAxis=+Z  RotationAngle=0.0  RotationArbitraryAxis=[0 0 1]  FollAlignAxisA=+X  BaseAlignAxisA=+Y  FollAlignAxisB=+Y  BaseAlignAxisB=+Z  RotationSequenceAxes=BaseAxes  RotationSequence=XYZ  RotationSequenceAngles=[0 0 0]  RotationSequenceAnglesUnits=rad  RotationMatrix=[1 0 0; 0 1 0; 0 0 1]  Quaternion=[1 0 0 0]
  joint2_OriginTransform1 : sm_lib/Frames and Transforms/Rigid Transform  TranslationMethod=Cartesian  TranslationStandardOffset=0  TranslationStandardOffsetUnits=m  TranslationStandardAxis=+Z  TranslationCartesianOffset=[a1 0 0]  TranslationCartesianOffsetUnits=m  TranslationROffset=0  TranslationROffsetUnits=m  TranslationZOffset=0  TranslationZOffsetUnits=m  TranslationThetaOffset=0  TranslationThetaOffsetUnits=deg  RotationMethod=RotationSequence  RotationAngleUnits=deg  RotationStandardAxis=+Z  RotationAngle=0.0  RotationArbitraryAxis=[0 0 1]  FollAlignAxisA=+X  BaseAlignAxisA=+Y  FollAlignAxisB=+Y  BaseAlignAxisB=+Z  RotationSequenceAxes=FollowerAxes  RotationSequence=XYZ  RotationSequenceAngles=[-pi/2 0 -pi/2]  RotationSequenceAnglesUnits=rad  RotationMatrix=[1 0 0; 0 1 0; 0 0 1]  Quaternion=[1 0 0 0]
  joint3_OriginTransform1 : sm_lib/Frames and Transforms/Rigid Transform  TranslationMethod=Cartesian  TranslationStandardOffset=0  TranslationStandardOffsetUnits=m  TranslationStandardAxis=+Z  TranslationCartesianOffset=[a2 0 0]  TranslationCartesianOffsetUnits=m  TranslationROffset=0  TranslationROffsetUnits=m  TranslationZOffset=0  TranslationZOffsetUnits=m  TranslationThetaOffset=0  TranslationThetaOffsetUnits=deg  RotationMethod=RotationSequence  RotationAngleUnits=deg  RotationStandardAxis=+Z  RotationAngle=0.0  RotationArbitraryAxis=[0 0 1]  FollAlignAxisA=+X  BaseAlignAxisA=+Y  FollAlignAxisB=+Y  BaseAlignAxisB=+Z  RotationSequenceAxes=FollowerAxes  RotationSequence=XYZ  RotationSequenceAngles=[0 0 0]  RotationSequenceAnglesUnits=rad  RotationMatrix=[1 0 0; 0 1 0; 0 0 1]  Quaternion=[1 0 0 0]
  joint4_OriginTransform1 : sm_lib/Frames and Transforms/Rigid Transform  TranslationMethod=Cartesian  TranslationStandardOffset=0  TranslationStandardOffsetUnits=m  TranslationStandardAxis=+Z  TranslationCartesianOffset=[a3 d4 0]  TranslationCartesianOffsetUnits=m  TranslationROffset=0  TranslationROffsetUnits=m  TranslationZOffset=0  TranslationZOffsetUnits=m  TranslationThetaOffset=0  TranslationThetaOffsetUnits=deg  RotationMethod=RotationSequence  RotationAngleUnits=deg  RotationStandardAxis=+Z  RotationAngle=0.0  RotationArbitraryAxis=[0 0 1]  FollAlignAxisA=+X  BaseAlignAxisA=+Y  FollAlignAxisB=+Y  BaseAlignAxisB=+Z  RotationSequenceAxes=FollowerAxes  RotationSequence=XYZ  RotationSequenceAngles=[-pi/2 0 0]  RotationSequenceAnglesUnits=rad  RotationMatrix=[1 0 0; 0 1 0; 0 0 1]  Quaternion=[1 0 0 0]
  link3 : sm_lib/Body Elements/File Solid  ExtGeomFileName=/home/jiehuang/Documents/Custom-Robot/Matlab_Study/Matlab2023Project/IntroductionBook/程序/XB4模型/XB4-3.STL  UnitType=Custom  ExtGeomFileUnits=mm  StepReaderType=HEX  ExportConvexHullGeometry=off  InertiaType=Custom  Mass=0  MassUnits=kg  CenterOfMass=[0 0 0]  CenterOfMassUnits=m  MomentsOfInertia=[0 0 0]  MomentsOfInertiaUnits=kg*m^2  ProductsOfInertia=[0 0 0]  ProductsOfInertiaUnits=kg*m^2  BasedOnType=Density  Density=1000  DensityUnits=kg/(m^3)  DoExposeReferenceFrame=on  SerializedFrames=<Frames/>  GraphicType=FromGeometry  MarkerShape=Sphere  MarkerSize=10  GraphicVisPropType=SimpleVisualProperties  GraphicDiffuseColor=[0.5 0.5 0.5]  GraphicSpecularColor=[0.5 0.5 0.5 1.0]  GraphicAmbientColor=[0.15 0.15 0.15 1.0]  GraphicEmissiveColor=[0.0 0.0 0.0 1.0]  GraphicShininess=75  GraphicOpacity=1.0
  F : PMIOPort  Side=Left
  F1 : PMIOPort  Port=2  Side=Right
  connections:
  Reference Frame/RConn1 -- joint3_OriginTransform1/RConn1 -- Inertia/RConn1 -- F/RConn1 -- joint4_OriginTransform1/LConn1
  F1/RConn1 -- joint4_OriginTransform1/RConn1
  joint1_OriginTransform1/RConn1 -- joint2_OriginTransform1/LConn1
  joint3_OriginTransform1/LConn1 -- joint2_OriginTransform1/RConn1
  link3/RConn1 -- joint1_OriginTransform1/LConn1

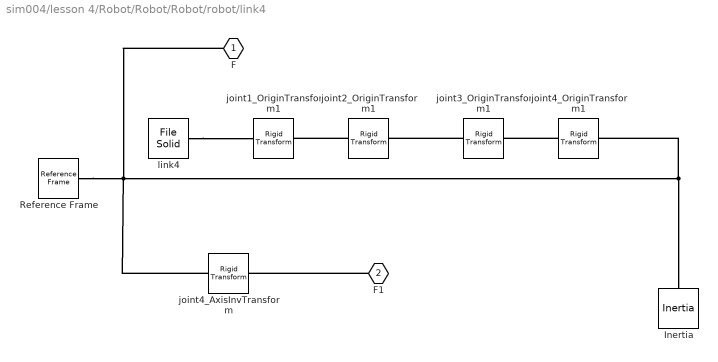
== system sim004/lesson 4/Robot/Robot/Robot/robot/link4 ==
  Inertia : sm_lib/Body Elements/Inertia  InertiaType=Custom  Mass=m4  MassUnits=kg  CenterOfMass=[mc41 mc42 mc43]  CenterOfMassUnits=m  MomentsOfInertia=[Ic411 Ic422 Ic433]  MomentsOfInertiaUnits=kg*m^2  ProductsOfInertia=[Ic423 Ic413 Ic412]  ProductsOfInertiaUnits=kg*m^2  GraphicType=Marker  MarkerShape=Inertia  MarkerSize=20  GraphicVisPropType=SimpleVisualProperties  GraphicDiffuseColor=[0.5 0.5 0.5]  GraphicSpecularColor=[0.5 0.5 0.5 1.0]  GraphicAmbientColor=[0.15 0.15 0.15 1.0]  GraphicEmissiveColor=[0.0 0.0 0.0 1.0]  GraphicShininess=75  GraphicOpacity=1.0
  Reference Frame : sm_lib/Frames and Transforms/Reference Frame
  joint1_OriginTransform1 : sm_lib/Frames and Transforms/Rigid Transform  TranslationMethod=Cartesian  TranslationStandardOffset=0  TranslationStandardOffsetUnits=m  TranslationStandardAxis=+Z  TranslationCartesianOffset=[0 0 d1]  TranslationCartesianOffsetUnits=m  TranslationROffset=0  TranslationROffsetUnits=m  TranslationZOffset=0  TranslationZOffsetUnits=m  TranslationThetaOffset=0  TranslationThetaOffsetUnits=deg  RotationMethod=RotationSequence  RotationAngleUnits=deg  RotationStandardAxis=+Z  RotationAngle=0.0  RotationArbitraryAxis=[0 0 1]  FollAlignAxisA=+X  BaseAlignAxisA=+Y  FollAlignAxisB=+Y  BaseAlignAxisB=+Z  RotationSequenceAxes=BaseAxes  RotationSequence=XYZ  RotationSequenceAngles=[0 0 0]  RotationSequenceAnglesUnits=rad  RotationMatrix=[1 0 0; 0 1 0; 0 0 1]  Quaternion=[1 0 0 0]
  joint2_OriginTransform1 : sm_lib/Frames and Transforms/Rigid Transform  TranslationMethod=Cartesian  TranslationStandardOffset=0  TranslationStandardOffsetUnits=m  TranslationStandardAxis=+Z  TranslationCartesianOffset=[a1 0 0]  TranslationCartesianOffsetUnits=m  TranslationROffset=0  TranslationROffsetUnits=m  TranslationZOffset=0  TranslationZOffsetUnits=m  TranslationThetaOffset=0  TranslationThetaOffsetUnits=deg  RotationMethod=RotationSequence  RotationAngleUnits=deg  RotationStandardAxis=+Z  RotationAngle=0.0  RotationArbitraryAxis=[0 0 1]  FollAlignAxisA=+X  BaseAlignAxisA=+Y  FollAlignAxisB=+Y  BaseAlignAxisB=+Z  RotationSequenceAxes=FollowerAxes  RotationSequence=XYZ  RotationSequenceAngles=[-pi/2 0 -pi/2]  RotationSequenceAnglesUnits=rad  RotationMatrix=[1 0 0; 0 1 0; 0 0 1]  Quaternion=[1 0 0 0]
  joint3_OriginTransform1 : sm_lib/Frames and Transforms/Rigid Transform  TranslationMethod=Cartesian  TranslationStandardOffset=0  TranslationStandardOffsetUnits=m  TranslationStandardAxis=+Z  TranslationCartesianOffset=[a2 0 0]  TranslationCartesianOffsetUnits=m  TranslationROffset=0  TranslationROffsetUnits=m  TranslationZOffset=0  TranslationZOffsetUnits=m  TranslationThetaOffset=0  TranslationThetaOffsetUnits=deg  RotationMethod=RotationSequence  RotationAngleUnits=deg  RotationStandardAxis=+Z  RotationAngle=0.0  RotationArbitraryAxis=[0 0 1]  FollAlignAxisA=+X  BaseAlignAxisA=+Y  FollAlignAxisB=+Y  BaseAlignAxisB=+Z  RotationSequenceAxes=FollowerAxes  RotationSequence=XYZ  RotationSequenceAngles=[0 0 0]  RotationSequenceAnglesUnits=rad  RotationMatrix=[1 0 0; 0 1 0; 0 0 1]  Quaternion=[1 0 0 0]
  joint4_AxisInvTransform : sm_lib/Frames and Transforms/Rigid Transform  TranslationMethod=Cartesian  TranslationStandardOffset=0  TranslationStandardOffsetUnits=m  TranslationStandardAxis=+Z  TranslationCartesianOffset=[0 0 0]  TranslationCartesianOffsetUnits=m  TranslationROffset=0  TranslationROffsetUnits=m  TranslationZOffset=0  TranslationZOffsetUnits=m  TranslationThetaOffset=0  TranslationThetaOffsetUnits=deg  RotationMethod=RotationSequence  RotationAngleUnits=rad  RotationStandardAxis=+Z  RotationAngle=1.570796  RotationArbitraryAxis=[0 1 0]  FollAlignAxisA=+X  BaseAlignAxisA=+Y  FollAlignAxisB=+Y  BaseAlignAxisB=+Z  RotationSequenceAxes=FollowerAxes  RotationSequence=XYZ  RotationSequenceAngles=[pi/2 0 0]  RotationSequenceAnglesUnits=rad  RotationMatrix=[1 0 0; 0 1 0; 0 0 1]  Quaternion=[1 0 0 0]
  joint4_OriginTransform1 : sm_lib/Frames and Transforms/Rigid Transform  TranslationMethod=Cartesian  TranslationStandardOffset=0  TranslationStandardOffsetUnits=m  TranslationStandardAxis=+Z  TranslationCartesianOffset=[a3 d4 0]  TranslationCartesianOffsetUnits=m  TranslationROffset=0  TranslationROffsetUnits=m  TranslationZOffset=0  TranslationZOffsetUnits=m  TranslationThetaOffset=0  TranslationThetaOffsetUnits=deg  RotationMethod=RotationSequence  RotationAngleUnits=deg  RotationStandardAxis=+Z  RotationAngle=0.0  RotationArbitraryAxis=[0 0 1]  FollAlignAxisA=+X  BaseAlignAxisA=+Y  FollAlignAxisB=+Y  BaseAlignAxisB=+Z  RotationSequenceAxes=FollowerAxes  RotationSequence=XYZ  RotationSequenceAngles=[-pi/2 0 0]  RotationSequenceAnglesUnits=rad  RotationMatrix=[1 0 0; 0 1 0; 0 0 1]  Quaternion=[1 0 0 0]
  link4 : sm_lib/Body Elements/File Solid  ExtGeomFileName=/home/jiehuang/Documents/Custom-Robot/Matlab_Study/Matlab2023Project/IntroductionBook/程序/XB4模型/XB4-4.STL  UnitType=Custom  ExtGeomFileUnits=mm  StepReaderType=HEX  ExportConvexHullGeometry=off  InertiaType=Custom  Mass=0  MassUnits=kg  CenterOfMass=[0 0 0]  CenterOfMassUnits=m  MomentsOfInertia=[0 0 0]  MomentsOfInertiaUnits=kg*m^2  ProductsOfInertia=[0 0 0]  ProductsOfInertiaUnits=kg*m^2  BasedOnType=Density  Density=1000  DensityUnits=kg/(m^3)  DoExposeReferenceFrame=on  SerializedFrames=<Frames/>  GraphicType=FromGeometry  MarkerShape=Sphere  MarkerSize=10  GraphicVisPropType=SimpleVisualProperties  GraphicDiffuseColor=[0.5 0.5 0.5]  GraphicSpecularColor=[0.5 0.5 0.5 1.0]  GraphicAmbientColor=[0.15 0.15 0.15 1.0]  GraphicEmissiveColor=[0.0 0.0 0.0 1.0]  GraphicShininess=75  GraphicOpacity=1.0
  F : PMIOPort  Side=Left
  F1 : PMIOPort  Port=2  Side=Right
  connections:
  Reference Frame/RConn1 -- Inertia/RConn1 -- joint4_OriginTransform1/RConn1 -- F/RConn1 -- joint4_AxisInvTransform/LConn1
  F1/RConn1 -- joint4_AxisInvTransform/RConn1
  joint4_OriginTransform1/LConn1 -- joint3_OriginTransform1/RConn1
  joint3_OriginTransform1/LConn1 -- joint2_OriginTransform1/RConn1
  joint2_OriginTransform1/LConn1 -- joint1_OriginTransform1/RConn1
  link4/RConn1 -- joint1_OriginTransform1/LConn1
